simulink model "F4_I2C_Master_WWDG"  (R2018b)
settings: Solver=FixedStepDiscrete  StartTime=0.0  StopTime=10.0  FixedStep=0.05  RelTol=1e-3  EnableMultiTasking=on
libraries: I2C_Lib x4, STM32_Config_Lib x1, WDG_Lib x1
settings Model: Creator=liprandd  LastModifiedBy=fenard1
settings DataIOCC: LimitDataPoints=on  SaveFormat=Array  SignalLoggingSaveFormat=ModelDataLogs
settings OptimizationCC: DefaultParameterBehavior=Inlined  DefaultUnderspecifiedDataType=single  PassReuseOutputArgsAs=Individual arguments  LifeSpan=1
settings DebuggingCC: UnderspecifiedInitializationDetection=Classic  MergeDetectMultiDrivingBlocksExec=none  SolverPrmCheckMsg=warning  MultiTaskDSMMsg=warning  MultiTaskCondExecSysMsg=none  UniqueDataStoreMsg=error  AllowSymbolicDim=off  StrictBusMsg=ErrorOnBusTreatedAsVector  SFUnexpectedBacktrackingDiag=warning  SFNoUnconditionalDefaultTransitionDiag=warning  SFUndirectedBroadcastEventsDiag=error  SFExecutionAtInitializationDiag=none
settings HardwareCC: ProdBitPerPointer=32  ProdBitPerSizeT=32  ProdBitPerPtrDiffT=32  ProdLargestAtomicInteger=Integer  ProdWordSize=32  ProdHWDeviceType=STMicroelectronics->STM32 32-bit Cortex-M
settings ModelReferenceCC: PropagateSignalLabelsOutOfModel=off
settings SFSimCC: SimUseLocalCustomCode=off  CompileTimeRecursionLimit=0  EnableRuntimeRecursion=off  MATLABDynamicMemAlloc=off
settings RTWCC: SystemTargetFile=stm32.tlc  TemplateMakefile=stm32.tmf  Description=stm32 (Embedded Target)  GenerateReport=on  RTWUseLocalCustomCode=off
settings CodeAppCC: IgnoreCustomStorageClasses=off  CustomSymbolStrType=$N$R$M  SimulinkBlockComments=off
settings STFCustomTargetCC: TargetLangStandard=C99 (ISO)  ParMdlRefBuildCompliant=on  IncludeMdlTerminateFcn=off  CombineOutputUpdateFcns=on  ERTCustomFileBanners=on  SupportNonFinite=off  SupportComplex=off  SupportContinuousTime=off  SupportNonInlinedSFcns=off  RemoveResetFunc=on  MATLABClassNameForMDSCustomization=Simulink.SoftwareTarget.ERTCustomization  SystemTargetFile=stm32.tlc
settings ERTTargetCC: TargetLangStandard=C99 (ISO)  MultiwordLength=2048  CompOptLevelCompliant=off  ConcurrentExecutionCompliant=off  IncludeMdlTerminateFcn=off  SupportNonFinite=off  SupportComplex=off  ModelStepFunctionPrototypeControlCompliant=off  CPPClassGenCompliant=off  UseToolchainInfoCompliant=off  ERTSrcFileBannerTemplate=sourceFileTemplate.cgt  ERTHdrFileBannerTemplate=sourceFileTemplate.cgt  ERTDataSrcFileTemplate=sourceFileTemplate.cgt  ERTDataHdrFileTemplate=sourceFileTemplate.cgt  ERTCustomFileTemplate=customRoutineProcess.tlc  ConvertIfToSwitch=off  SuppressUnreachableDefaultCases=off  EnableSignedLeftShifts=off  EnableSignedRightShifts=off
settings ConfigComp: CovMetricSettings=dw  CovHtmlReporting=on  CovSaveCumulativeToWorkspaceVar=on  CovSaveSingleToWorkspaceVar=on  CovExternalEMLEnable=off  CovSFcnEnable=off

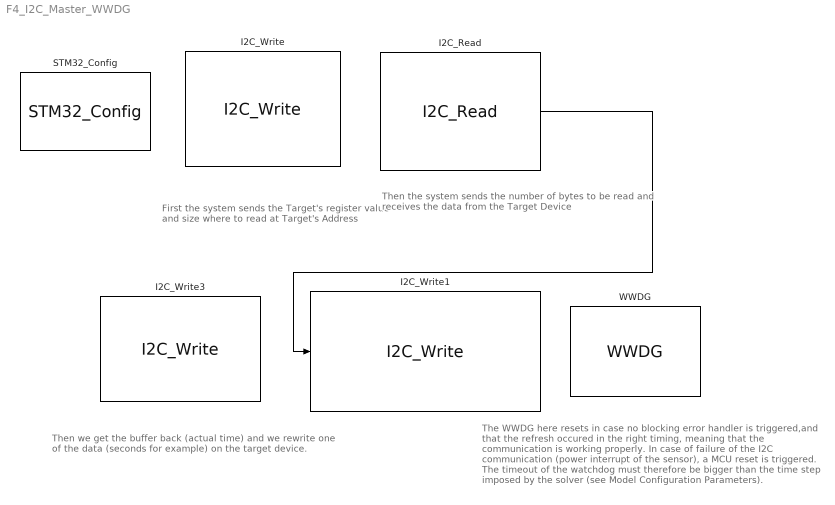
== system F4_I2C_Master_WWDG ==
  note: First the system sends the
      | Target's register value and size
      | where to read at Target's Address
  note: Then the system sends the
      | number of bytes to be read and
      | receives the data from the Target Device
  note: Then we get the buffer back (actual time)
      | and we rewrite one of the data (seconds
      | for example) on the target device.
  note: The WWDG here resets in case no blocking
      | error handler is triggered,and that the refresh
      | occured in the right timing, meaning that the
      | communication is working properly. In case
      | of failure of the I2C communication (power
      | interrupt of the sensor), a MCU reset is triggered.
      | The timeout of the watchdog must therefore be
      | bigger than the time step imposed by the solver
      | (see Model Configuration Parameters).
  I2C_Read : I2C_Lib/I2C_Read  Priority=1  i2cx=I2C1  Device_Mode=MASTER  Device_Address=62  i2c_Mode=DMA_RX_TX  Target_Address=0  handler=hi2c1  Buffer_Size=3  Timeout=50  TimeoutValue=2.5  Enable_Output=on  Error=off  CallBack=off
      settings: SourceProductName=Target Support Package - STM32 Adapter
  I2C_Write : I2C_Lib/I2C_Write  Priority=0  i2cx=I2C1  Device_Mode=MASTER  Target_Address=160  Target_Register=2  Enable_Input=off  Data_str={2}  i2c_Mode=DMA_RX_TX  Buffer_Size=1  handler=hi2c1  Timeout=50  TimeoutValue=2.5  Error=off  CallBack=off
      settings: SourceProductName=Target Support Package - STM32 Adapter
  I2C_Write1 : I2C_Lib/I2C_Write  Priority=3  i2cx=I2C1  Device_Mode=MASTER  Target_Address=160  Target_Register=3  Enable_Input=on  Data_str={18,0x02,0x09,0x13}  i2c_Mode=DMA_RX_TX  Buffer_Size=3  handler=hi2c1  Timeout=50  TimeoutValue=2.5  Error=off  CallBack=off
      settings: SourceProductName=Target Support Package - STM32 Adapter
  I2C_Write3 : I2C_Lib/I2C_Write  Priority=2  i2cx=I2C1  Device_Mode=MASTER  Target_Address=160  Target_Register=2  Enable_Input=off  Data_str={2}  i2c_Mode=DMA_RX_TX  Buffer_Size=1  handler=hi2c1  Timeout=50  TimeoutValue=2.5  Error=off  CallBack=off
      settings: SourceProductName=Target Support Package - STM32 Adapter
  STM32_Config : STM32_Config_Lib/STM32_Config  Project_Path=.\  Config_File=F4_I2C_Master_WWDG.ioc  MCU_Name=STM32F429ZITx
      settings: SourceProductName=Target Support Package - STM32 Adapter
  WWDG : WDG_Lib/WWDG  Window=70  Custom_Window=off  Counter=127  Custom_Counter=off  Period=5.242880e+01ms  t_min=4.669440e+01ms  t_max=5.242880e+01ms
      settings: SourceProductName=Target Support Package - STM32 Adapter
  wires:
  I2C_Read/1 -> I2C_Write1/1
